simulink model "LW_ctrl_241029_1"  (R2024b)
settings: Solver=ode4  StartTime=0.0  StopTime=inf  FixedStep=0.005  RelTol=1e-3  EnableMultiTasking=on
StartFcn:
  | %timestart = cputime;
StopFcn:
  | %dt = cputime - timestart
undefined symbols (not defined in the file or in its folder): AttCtrl_cycle, ControlMode, DEG2RAD, Earth, FlightMode, LW_ACRO_P_MAX, LW_ACRO_R_MAX, LW_ACRO_Y_MAX, LW_AERO_C0, LW_AERO_C1, LW_AERO_Y0, LW_ANGLE, LW_DMZ0, LW_DMZ_MIN, LW_LAT_CIRCLE, LW_MAN_PITCH_MAX, LW_MAN_ROLL_MAX, LW_MASS, LW_OB_CIRCLE_R, LW_OB_CIRCLE_V, LW_OB_CIRCLE_W, LW_OB_TYPE, LW_REX_YAW, LW_SERVOL_MAX, LW_SERVOR_MAX, LW_TEST_DTXY, LW_TEST_DTZ, LW_THR_HOVER, LW_WZ_MAX, LW_X_ACCEL_MAX, LW_X_ACCEL_MIN, LW_X_FF, LW_X_JERK_MAX, LW_X_P, LW_X_VEL_MAX, LW_Y_ACCEL_MAX, LW_Y_ACCEL_MIN, LW_Y_FF, LW_Y_JERK_MAX, LW_Y_P, LW_Y_VEL_MAX, LW_YAW_KAD, LW_YAW_KAP, LW_Z_ACCEL_LOW, LW_Z_ACCEL_UP, LW_Z_FF, LW_Z_JERK_MAX, LW_Z_P, LW_Z_VEL_MAX_UP, Map_xoffset, Map_yoffset, Map_zoffset, MAX_wdotx, MAX_wdoty, MAX_wdotz, Mixer_cycle, ModelParam_AccelMax, ModelParam_DelayAtt, ModelParam_DelayOmega, ModelParam_DelayPos ... (+59)
libraries: pixhawk_slib_uORB_RW x15, simulink x7, slpidlib x6, dspfdesign x6, dspstat3 x5, aerolibnav x4, pixhawk_slib_sensors_actuators x3, aerolibtransform2 x3, etargetslib x2, pixhawk_slib_rfly x1, aerolibatmos2 x1, slrealtimeiplib x1
(part 1 of 6)
Description:
  | 20241104
  | 1.加入PX4中weather vane方法，并可以与偏航导纳相互切换，用于对比实验。
  | 2.加入没有进入定点以及手动控制偏航时对偏航导纳期望进行重置。
  |   进行了实飞测试，结果正常。
  | 
  | 20241030
  | 1.增加偏航导纳控制，加入4个偏航导纳控制相关的可调参数，并进行仿真测试。
  |   将力矩扰动估计放到状态更新模块中。
  | 2.修改模型加入φ理论气动力矩。
  | 3.位置控制输出部分增加姿态角速率，并在角速率控制部分加入手动模式下位置控制角速率前馈。
  | 20240905
  | 1.舵面滤波，增加舵面高速时的权重
  | 20240831
  | 1.加入舵面参数辨识的代码，修改混控制部分输出。
  |   设置参数为不使用舵面，在进入平飞状态时给一个固定的舵面角度。
  | 2.增加更多的直线轨迹，目前包括3,6,10,12,13,14,15,16,17,18,20
  | 20240826
  | 1.加入状态重置处理，包括控制器中、扰动估计中、offboard中
  | 2.修改混控器权重系数，优化空速较小时舵面变化大的问题。
  |   加入分别计算舵面和旋翼的代码。
  | 3.在6C和Pixhawk4中进行了实时性测试，250Hz都能实时运行；400Hz6C可以。
  | 
  | 关闭遥控器失联的处理；
  | 关闭acro模式；
  | 加入前馈系数；
  | 内置传感器中加入tfsensor启动指令；--20221019
  | 
  | 修改姿态控制逻辑，姿态误差在body系下求取，得到期望角速度之后转到lifting wing frame。--20221022
settings Model: Creator=Mr Wang  LastModifiedBy=bhcxq
settings SolverCC: AlgebraicLoopSolver=TrustRegion  PositivePriorityOrder=on  AutoInsertRateTranBlk=on
settings DataIOCC: ReturnWorkspaceOutputs=off
settings OptimizationCC: DefaultParameterBehavior=Inlined  MemcpyThreshold=128  MaxStackSize=128  EfficientTunableParamExpr=on
settings DebuggingCC: MergeDetectMultiDrivingBlocksExec=none  MultiTaskCondExecSysMsg=none  ParameterTunabilityLossMsg=error  UnconnectedInputMsg=warning  UnconnectedOutputMsg=warning  UnconnectedLineMsg=warning  AssertControl=DisableAll  ArithmeticOperatorsInVariantConditions=warning
settings HardwareCC: ProdBitPerPointer=32  ProdBitPerSizeT=32  ProdBitPerPtrDiffT=32  ProdLargestAtomicInteger=Long  ProdLargestAtomicFloat=Double  ProdWordSize=32  ProdHWDeviceType=ARM Compatible->ARM Cortex
settings ModelReferenceCC: EnableRefExpFcnMdlSchedulingChecks=on
settings SFSimCC: SimUseLocalCustomCode=off  MATLABDynamicMemAlloc=off  CustomCodeUndefinedFunction=UseInterfaceOnly
settings RTWCC: Description=Embedded Coder  SystemTargetFile=ert.tlc  HardwareBoard=Pixhawk PX4  TLCOptions="-aInlineSetEventsForThisBaseRateFcn=TLC_FALSE -aSuppressMultiTaskScheduler=TLC_FALSE  -aRateBasedStepFcn=0"  TemplateMakefile=ert_default_tmf  GenerateReport=on  RTWUseLocalCustomCode=off  CustomSource=px4_simulink_app_params.c  Toolchain=Pixhawk Toolchain  IncludeHyperlinkInReport=on  LaunchReport=on  CodeExecutionProfiling=on  CodeProfilingInstrumentation=detailed  GenerateTraceInfo=on  GenerateTraceReport=on  GenerateTraceReportSl=on  GenerateTraceReportSf=on  GenerateTraceReportEml=on  GPUComputeCapability=3.5  DLArmComputeVersion=19.05
settings CodeAppCC: ForceParamTrailComments=on  IgnoreCustomStorageClasses=off  OperatorAnnotations=on  SimulinkDataObjDesc=on  SFDataObjDesc=on  MATLABFcnDesc=on  InsertBlockDesc=on  StateflowObjectComments=on  MATLABSourceComments=on
settings ERTTargetCC: MultiwordLength=2048  SupportContinuousTime=on  SupportVariableSizeSignals=on  ExtModeTransport=1  ExtModeMexFile=ext_serial_win32_comm  ExtModeMexArgs=1 3 115200 10  InlinedParameterPlacement=Hierarchical  ERTCustomFileTemplate=px4_codertarget_file_process.tlc  ConvertIfToSwitch=off  DynamicArrayContainerType=coder::array
settings ConfigComp: PSEnableModelRefIgnoreList=off  PSModelRefMinMaxVerif=CheckAndConstrain  PSAutoStubLUT=on

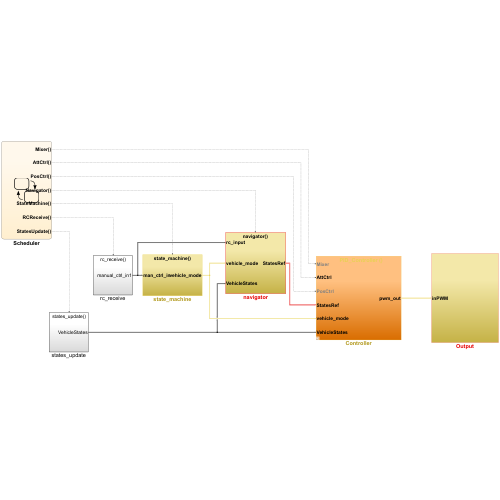
[thumbnail: Simulink's stored preview of the top-level diagram]
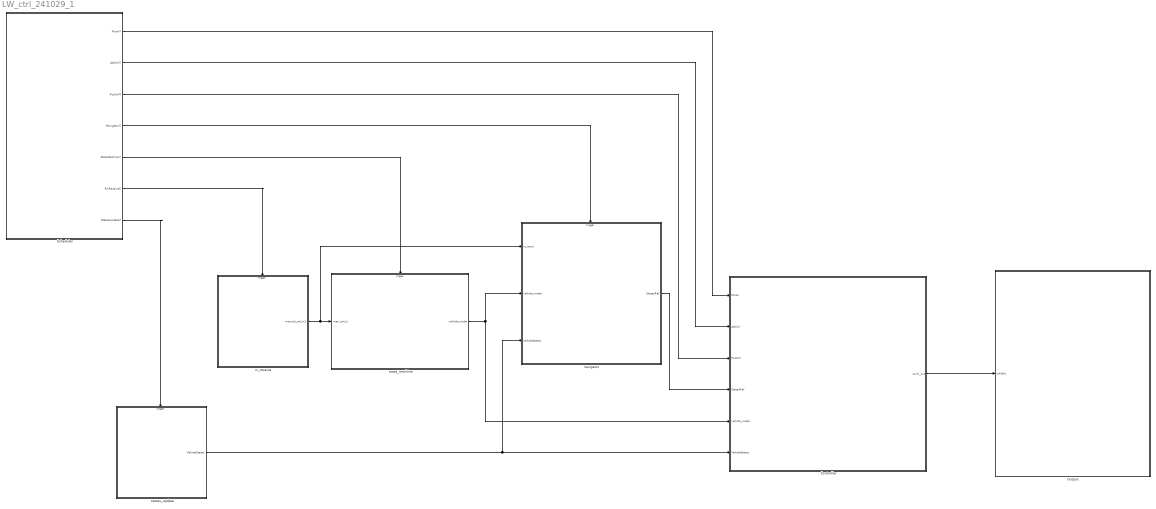
== system LW_ctrl_241029_1 ==
  Controller : Subsystem  Variant=on
  Output : Subsystem  Priority=8
  Scheduler : Stateflow chart  Priority=1  TreatAsAtomicUnit=on
  navigator : Subsystem  Priority=5
  rc_receive : Subsystem  Priority=3
  state_machine : Subsystem  Priority=4
  states_update : Subsystem  Priority=2
  wires:
  state_machine/1(vehicle_mode) -> Controller/5(vehicle_mode), navigator/2(vehicle_mode)
  rc_receive/1(manual_ctrl_in1) -> state_machine/1(man_ctrl_in), navigator/1(rc_input)
  states_update/1(VehicleStates) -> Controller/6(VehicleStates), navigator/3(VehicleStates)
  Scheduler/1(Mixer()) -> Controller/1(Mixer)
  Scheduler/2(AttCtrl()) -> Controller/2(AttCtrl)
  Scheduler/3(PosCtrl()) -> Controller/3(PosCtrl)
  Scheduler/7(StatesUpdate()) -> states_update/Trigger
  Scheduler/6(RCReceive()) -> rc_receive/Trigger
  Scheduler/5(StateMachine()) -> state_machine/Trigger
  Scheduler/4(Navigator()) -> navigator/Trigger
  navigator/1(StatesRef) -> Controller/4(StatesRef)
  Controller/1(pwm_out) -> Output/1(inPWM)

== system LW_ctrl_241029_1/Controller ==
  note: 1) Add Subsystem or Model blocks as valid variant choices.
      | 2) You cannot connect blocks at this level. At simulation, connectivity is automatically
      | determined, based on the active variant and port name matching.
  Mixer : Inport
  AttCtrl : Inport  Port=2
  PosCtrl : Inport  Port=3
  StatesRef : Inport  Port=4
  vehicle_mode : Inport  Port=5
  VehicleStates : Inport  Port=6
  PID_Controller : Subsystem  VariantControl=Controller_Switch <= 0.5
  pwm_out : Outport

== system LW_ctrl_241029_1/Output ==
  inPWM : Inport
  OutputSelect : Subsystem  Variant=on
  wires:
  inPWM/1 -> OutputSelect/1(inPWM)

== system LW_ctrl_241029_1/navigator ==
  rc_input : Inport
  vehicle_mode : Inport  Port=2
  VehicleStates : Inport  Port=3
  navigator : TriggerPort  TriggerType=function-call  VariantControl=Variant
  Bus Selector : BusSelector  OutputSignals=flight_mode
  StatesRefBus : BusCreator  Inputs=2
  Switch Case : SwitchCase  CaseConditions={FlightMode.PILOT, FlightMode.AUTO, FlightMode.OFFBOARD}  ShowDefaultCase=off
  Terminator : Terminator
  Terminator1 : Terminator
  logger : Subsystem  Variant=on
  navigator_manual : Subsystem  TreatAsAtomicUnit=on
  navigator_offboard : Subsystem  TreatAsAtomicUnit=on
  StatesRef : Outport  VectorParamsAs1DForOutWhenUnconnected=off
  tag scope: log_n_manual_ref=global, log_n_offboard_ref=global
  wires:
  Bus Selector/1 -> navigator_offboard/2(flight_mode), Switch Case/1  "<flight_mode>"
  Switch Case/1 -> navigator_manual/Action
  rc_input/1 -> navigator_offboard/3(RC_input), navigator_manual/1(rc_input)
  navigator_offboard/1(offboard_ref) -> [log_n_offboard_ref], StatesRefBus/2  "offboard"
  navigator_manual/1(manual_ref) -> [log_n_manual_ref], StatesRefBus/1  "manual"
  vehicle_mode/1 -> Bus Selector/1  "vehicle_mode"
  VehicleStates/1 -> navigator_offboard/1(VehicleStates)
  Switch Case/2 -> Terminator/1
  Switch Case/3 -> Terminator1/1
  StatesRefBus/1 -> StatesRef/1

== system LW_ctrl_241029_1/rc_receive ==
  rc_receive : TriggerPort  TriggerType=function-call  VariantControl=Variant
  manual_ctrl_in : Subsystem  Variant=on
  manual_ctrl_in1 : Outport
  wires:
  manual_ctrl_in/1(manual_ctrl_in) -> manual_ctrl_in1/1

== system LW_ctrl_241029_1/state_machine ==
  man_ctrl_in : Inport
  state_machine : TriggerPort  TriggerType=function-call  VariantControl=Variant
  Bus Creator : BusCreator  Inputs=3
  Bus Selector : BusSelector  OutputSignals=AU8,RC_Lost,AU5,AU7,AU6
  Bus Selector1 : BusSelector  OutputSignals=armed
  MATLAB Function3 : MATLAB Function  TreatAsAtomicUnit=on
  MATLAB Function4 : MATLAB Function  TreatAsAtomicUnit=on
  logger : Subsystem  Variant=on
  uORB Read Function-Call Trigger : pixhawk_slib_uORB_RW/uORB Read Function-Call Trigger  uORB_Topic_str='actuator_armed'  BusObjVar=Bus: actuator_armed_SL  uORB_Interval=4  AsyncOutput=off  Fcn_call_select=Generate Function Call Signal  TaskName='Task1'  Poll_timeout=-1  Ts=-1
      settings: SourceProductName=uORB Read / Write Blocks
  vehicle_mode : Outport  VectorParamsAs1DForOutWhenUnconnected=off
  tag scope: log_sm_vehicle_mode=global
  wires:
  man_ctrl_in/1 -> Bus Selector/1
  Bus Selector/3 -> MATLAB Function4/1(ch5)  "<AU5>"
  Bus Selector/2 -> MATLAB Function4/4(RC_Lost)  "<RC_Lost>"
  MATLAB Function4/2(flight_mode) -> Bus Creator/1
  Bus Selector/4 -> MATLAB Function4/2(ch7)  "<AU7>"
  Bus Selector/5 -> MATLAB Function3/1(ch6)  "<AU6>"
  Bus Creator/1 -> [log_sm_vehicle_mode], vehicle_mode/1
  MATLAB Function3/1(arm) -> Bus Creator/3  "arm"
  Bus Selector/1 -> MATLAB Function4/3(ch8)  "<AU8>"
  MATLAB Function4/1(ctrl_mode) -> Bus Creator/2  "ctrl_mode"
  uORB Read Function-Call Trigger/1 -> Bus Selector1/1
  Bus Selector1/1 -> MATLAB Function3/2(armed), MATLAB Function4/5(armed)  "<armed>"

== system LW_ctrl_241029_1/states_update ==
  states_update : TriggerPort  TriggerType=function-call  VariantControl=Variant
  Bus Creator : BusCreator  Inputs=8
  vehicle_local_position : Subsystem  Variant=on
  VehicleStates : Outport
  wires:
  vehicle_local_position/3(vehicle_attitude) -> Bus Creator/3  "vehicle_attitude"
  vehicle_local_position/2(airspeed) -> Bus Creator/2  "airspeed"
  vehicle_local_position/1(vehicle_local_position) -> Bus Creator/1  "vehicle_local_position"
  Bus Creator/1 -> VehicleStates/1
  vehicle_local_position/4(vehicle_global_position) -> Bus Creator/4  "vehicle_global_position"
  vehicle_local_position/5(battery_status) -> Bus Creator/5  "battery_status"
  vehicle_local_position/6(T_limit) -> Bus Creator/6  "T_limit"
  vehicle_local_position/7(sensor_imu) -> Bus Creator/7  "sensor_imu"
  vehicle_local_position/8(states_flag) -> Bus Creator/8  "states_flag"

== system LW_ctrl_241029_1/Controller/PID_Controller ==
  StatesRef : Inport
  vehicle_mode : Inport  Port=2
  VehicleStates : Inport  Port=3
  AttCtrl : TriggerPort  TriggerType=function-call  VariantControl=Variant
  PID_Controller : Subsystem  VariantControl=Controller_Switch <= 1.5 && Controller_Switch >= 0.5
  pwm_out : Outport
  wires:
  StatesRef/1 -> PID_Controller/1(StatesRef)
  PID_Controller/1(pwm_out) -> pwm_out/1
  vehicle_mode/1 -> PID_Controller/2(vehicle_mode)
  VehicleStates/1 -> PID_Controller/3(VehicleStates)

== system LW_ctrl_241029_1/Output/OutputSelect ==
  note: 1) Add Subsystem or Model blocks as valid variant choices.
      | 2) You cannot connect blocks at this level. At simulation, connectivity is automatically
      | determined, based on the active variant and port name matching.
  inPWM : Inport
  FLY : Subsystem  VariantControl=VSS_PROCEDURE_FLY
  HIL : Subsystem  VariantControl=VSS_PROCEDURE_HIL
  Sim : Subsystem  TreatAsAtomicUnit=on  VariantControl=VSS_PROCEDURE_SIM

== system LW_ctrl_241029_1/navigator/logger ==
  HIL&FLY : Subsystem  VariantControl=VSS_PROCEDURE_HIL_FLY
  Sim : Subsystem  VariantControl=VSS_PROCEDURE_SIM

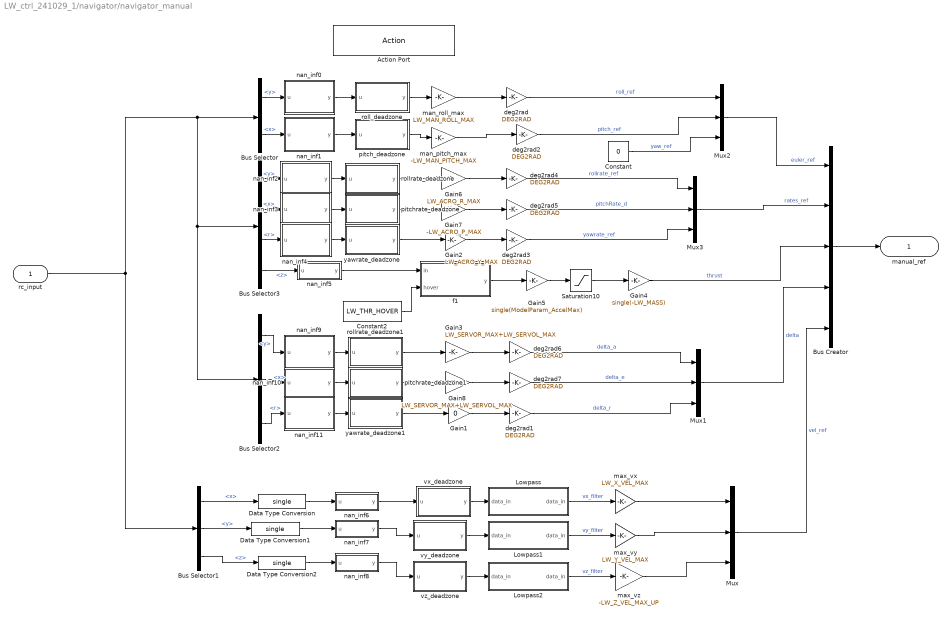
== system LW_ctrl_241029_1/navigator/navigator_manual ==
  rc_input : Inport
  Action Port : ActionPort  ActionPortLabel=case [ PILOT ]:
  Bus Creator : BusCreator  Inputs=5
  Bus Selector : BusSelector  OutputSignals=y,x
  Bus Selector1 : BusSelector  OutputSignals=x,y,z
  Bus Selector2 : BusSelector  OutputSignals=y,x,r
  Bus Selector3 : BusSelector  OutputSignals=y,x,r,z
  Constant : Constant  Value=0  OutDataTypeStr=single
  Constant2 : Constant  Value=LW_THR_HOVER
  Data Type Conversion : DataTypeConversion  OutDataTypeStr=single  SaturateOnIntegerOverflow=off  RndMeth=Floor
  Data Type Conversion1 : DataTypeConversion  OutDataTypeStr=single  SaturateOnIntegerOverflow=off  RndMeth=Floor
  Data Type Conversion2 : DataTypeConversion  OutDataTypeStr=single  SaturateOnIntegerOverflow=off  RndMeth=Floor
  Gain1 : Gain  Gain=0
  Gain2 : Gain  Gain=LW_ACRO_Y_MAX
  Gain3 : Gain  Gain=LW_SERVOR_MAX+LW_SERVOL_MAX  OutDataTypeStr=Inherit: Inherit via back propagation
  Gain4 : Gain  Gain=single(-LW_MASS)
  Gain5 : Gain  Gain=single(ModelParam_AccelMax)
  Gain6 : Gain  Gain=LW_ACRO_R_MAX  OutDataTypeStr=Inherit: Inherit via back propagation
  Gain7 : Gain  Gain=-LW_ACRO_P_MAX  OutDataTypeStr=Inherit: Inherit via back propagation
  Gain8 : Gain  Gain=LW_SERVOR_MAX+LW_SERVOL_MAX  OutDataTypeStr=Inherit: Inherit via back propagation
  Lowpass : MATLAB Function  TreatAsAtomicUnit=on
  Lowpass1 : MATLAB Function  TreatAsAtomicUnit=on
  Lowpass2 : MATLAB Function  TreatAsAtomicUnit=on
  Mux{,1..3} (4 alike) : Mux  Inputs=3
  Saturation10 : Saturate  UpperLimit=single(5+ModelParam_envGravityAcc)  LowerLimit=0
  deg2rad{,1..7} (8 alike) : Gain  Gain=DEG2RAD
  f1 : MATLAB Function  TreatAsAtomicUnit=on
  man_pitch_max : Gain  Gain=-LW_MAN_PITCH_MAX  OutDataTypeStr=Inherit: Inherit via back propagation
  man_roll_max : Gain  Gain=LW_MAN_ROLL_MAX  OutDataTypeStr=Inherit: Inherit via back propagation
  max_vx : Gain  Gain=LW_X_VEL_MAX  OutDataTypeStr=Inherit: Inherit via back propagation
  max_vy : Gain  Gain=LW_Y_VEL_MAX  OutDataTypeStr=Inherit: Inherit via back propagation
  max_vz : Gain  Gain=-LW_Z_VEL_MAX_UP  OutDataTypeStr=Inherit: Inherit via back propagation
  nan_inf0 : MATLAB Function  TreatAsAtomicUnit=on
  nan_inf1 : MATLAB Function  TreatAsAtomicUnit=on
  nan_inf10 : MATLAB Function  TreatAsAtomicUnit=on
  nan_inf11 : MATLAB Function  TreatAsAtomicUnit=on
  nan_inf2 : MATLAB Function  TreatAsAtomicUnit=on
  nan_inf3 : MATLAB Function  TreatAsAtomicUnit=on
  nan_inf4 : MATLAB Function  TreatAsAtomicUnit=on
  nan_inf5 : MATLAB Function  TreatAsAtomicUnit=on
  nan_inf6 : MATLAB Function  TreatAsAtomicUnit=on
  nan_inf7 : MATLAB Function  TreatAsAtomicUnit=on
  nan_inf8 : MATLAB Function  TreatAsAtomicUnit=on
  nan_inf9 : MATLAB Function  TreatAsAtomicUnit=on
  pitch_deadzone : MATLAB Function  TreatAsAtomicUnit=on
  pitchrate_deadzone : MATLAB Function  TreatAsAtomicUnit=on
  pitchrate_deadzone1 : MATLAB Function  TreatAsAtomicUnit=on
  roll_deadzone : MATLAB Function  TreatAsAtomicUnit=on
  rollrate_deadzone : MATLAB Function  TreatAsAtomicUnit=on
  rollrate_deadzone1 : MATLAB Function  TreatAsAtomicUnit=on
  vx_deadzone : MATLAB Function  TreatAsAtomicUnit=on
  vy_deadzone : MATLAB Function  TreatAsAtomicUnit=on
  vz_deadzone : MATLAB Function  TreatAsAtomicUnit=on
  yawrate_deadzone : MATLAB Function  TreatAsAtomicUnit=on
  yawrate_deadzone1 : MATLAB Function  TreatAsAtomicUnit=on
  manual_ref : Outport
  wires:
  Gain4/1 -> Bus Creator/3  "thrust"
  man_roll_max/1 -> deg2rad/1
  Gain2/1 -> deg2rad3/1
  man_pitch_max/1 -> deg2rad2/1
  Bus Creator/1 -> manual_ref/1
  Bus Selector3/3 -> nan_inf4/1(u)  "<r>"
  deg2rad/1 -> Mux2/1  "roll_ref"
  Bus Selector3/4 -> nan_inf5/1(u)  "<z>"
  deg2rad2/1 -> Mux2/2  "pitch_ref"
  Bus Selector/2 -> nan_inf1/1(u)  "<x>"
  Bus Selector/1 -> nan_inf0/1(u)  "<y>"
  deg2rad3/1 -> Mux3/3  "yawrate_ref"
  Bus Selector1/3 -> Data Type Conversion2/1  "<z>"
  Data Type Conversion/1 -> nan_inf6/1(u)
  Data Type Conversion2/1 -> nan_inf8/1(u)
  Bus Selector1/2 -> Data Type Conversion1/1  "<y>"
  Data Type Conversion1/1 -> nan_inf7/1(u)
  Bus Selector1/1 -> Data Type Conversion/1  "<x>"
  max_vz/1 -> Mux/3
  max_vx/1 -> Mux/1
  max_vy/1 -> Mux/2
  Mux/1 -> Bus Creator/5  "vel_ref"
  Constant/1 -> Mux2/3  "yaw_ref"
  Mux2/1 -> Bus Creator/1  "euler_ref"
  deg2rad4/1 -> Mux3/1  "rollrate_ref"
  Gain6/1 -> deg2rad4/1
  Bus Selector3/1 -> nan_inf2/1(u)  "<y>"
  deg2rad5/1 -> Mux3/2  "pitchRate_d"
  Gain7/1 -> deg2rad5/1
  Bus Selector3/2 -> nan_inf3/1(u)  "<x>"
  Mux3/1 -> Bus Creator/2  "rates_ref"
  nan_inf5/1(y) -> f1/1(in)
  Gain5/1 -> Saturation10/1
  Saturation10/1 -> Gain4/1
  roll_deadzone/1(y) -> man_roll_max/1
  pitch_deadzone/1(y) -> man_pitch_max/1
  rollrate_deadzone/1(y) -> Gain6/1
  pitchrate_deadzone/1(y) -> Gain7/1
  yawrate_deadzone/1(y) -> Gain2/1
  vx_deadzone/1(y) -> Lowpass/1("data_in ")
  vy_deadzone/1(y) -> Lowpass1/1("data_in ")
  vz_deadzone/1(y) -> Lowpass2/1("data_in ")
  nan_inf0/1(y) -> roll_deadzone/1(u)
  nan_inf1/1(y) -> pitch_deadzone/1(u)
  nan_inf2/1(y) -> rollrate_deadzone/1(u)
  nan_inf3/1(y) -> pitchrate_deadzone/1(u)
  nan_inf4/1(y) -> yawrate_deadzone/1(u)
  nan_inf6/1(y) -> vx_deadzone/1(u)
  nan_inf7/1(y) -> vy_deadzone/1(u)
  nan_inf8/1(y) -> vz_deadzone/1(u)
  f1/1(y) -> Gain5/1
  Constant2/1 -> f1/2(hover)
  nan_inf11/1(y) -> yawrate_deadzone1/1(u)
  nan_inf10/1(y) -> pitchrate_deadzone1/1(u)
  nan_inf9/1(y) -> rollrate_deadzone1/1(u)
  yawrate_deadzone1/1(y) -> Gain1/1
  pitchrate_deadzone1/1(y) -> Gain8/1
  rollrate_deadzone1/1(y) -> Gain3/1
  Mux1/1 -> Bus Creator/4  "delta"
  Bus Selector2/2 -> nan_inf10/1(u)  "<x>"
  Gain8/1 -> deg2rad7/1
  deg2rad7/1 -> Mux1/2  "delta_e"
  Bus Selector2/1 -> nan_inf9/1(u)  "<y>"
  Gain3/1 -> deg2rad6/1
  deg2rad6/1 -> Mux1/1  "delta_a"
  deg2rad1/1 -> Mux1/3  "delta_r"
  Bus Selector2/3 -> nan_inf11/1(u)  "<r>"
  Gain1/1 -> deg2rad1/1
  rc_input/1 -> Bus Selector1/1, Bus Selector2/1, Bus Selector3/1, Bus Selector/1
  Lowpass/1(data_in) -> max_vx/1  "vx_filter"
  Lowpass1/1(data_in) -> max_vy/1  "vy_filter"
  Lowpass2/1(data_in) -> max_vz/1  "vz_filter"

== system LW_ctrl_241029_1/navigator/navigator_offboard ==
  VehicleStates : Inport
  flight_mode : Inport  Port=2
  RC_input : Inport  Port=3
  Bus Selector1 : BusSelector  OutputSignals=AU8
  Bus Selector2 : BusSelector  OutputSignals=vehicle_local_position.timestamp,vehicle_local_position.vehicle_local_pos,vehicle_local_position.vehicle_local_vel,vehicle_attitude.quat,airspeed.v_wind
  Data Type Conversion : DataTypeConversion  OutDataTypeStr=single  SaturateOnIntegerOverflow=off  RndMeth=Floor
  Gain : Gain  Gain=1.0e-6
  task select : Subsystem
  offboard_ref : Outport  OutDataTypeStr=Bus: offboard_bus
  wires:
  Bus Selector2/2 -> task select/3(pos)  "<vehicle_local_pos>"
  Bus Selector2/3 -> task select/4(vel)  "<vehicle_local_vel>"
  Bus Selector2/4 -> task select/5(q)  "<quat>"
  Data Type Conversion/1 -> task select/1(timestamp)
  VehicleStates/1 -> Bus Selector2/1
  flight_mode/1 -> task select/2(flight_mode)
  Gain/1 -> Data Type Conversion/1
  Bus Selector2/5 -> task select/7(v_wind)  "<v_wind>"
  Bus Selector2/1 -> Gain/1  "<timestamp>"
  RC_input/1 -> Bus Selector1/1
  Bus Selector1/1 -> task select/6(CH8)  "<AU8>"
  task select/1(offboard_ref) -> offboard_ref/1

== system LW_ctrl_241029_1/rc_receive/manual_ctrl_in ==
  HIL&FLY V1.13.3 : Subsystem  VariantControl=VSS_PROCEDURE_HIL_FLY_V1_13
  Sim : Subsystem  VariantControl=VSS_PROCEDURE_SIM
  manual_ctrl_in : Outport  VectorParamsAs1DForOutWhenUnconnected=off

== system LW_ctrl_241029_1/state_machine/logger ==
  HIL&FLY : Subsystem  VariantControl=VSS_PROCEDURE_HIL_FLY
  Sim : Subsystem  VariantControl=VSS_PROCEDURE_SIM

== system LW_ctrl_241029_1/states_update/vehicle_local_position ==
  HIL&FLY V1.13.3 : Subsystem  VariantControl=VSS_PROCEDURE_HIL_FLY_V1_13
  Sim : Subsystem  VariantControl=VSS_PROCEDURE_SIM
  vehicle_local_position : Outport  VectorParamsAs1DForOutWhenUnconnected=off
  airspeed : Outport  Port=2  VectorParamsAs1DForOutWhenUnconnected=off
  vehicle_attitude : Outport  Port=3  VectorParamsAs1DForOutWhenUnconnected=off
  vehicle_global_position : Outport  Port=4  OutDataTypeStr=Bus: vehicle_global_position_bus  VectorParamsAs1DForOutWhenUnconnected=off
  battery_status : Outport  Port=5  OutDataTypeStr=Bus: battery_status_bus  VectorParamsAs1DForOutWhenUnconnected=off
  T_limit : Outport  Port=6  VectorParamsAs1DForOutWhenUnconnected=off
  sensor_imu : Outport  Port=7  VectorParamsAs1DForOutWhenUnconnected=off
  states_flag : Outport  Port=8  VectorParamsAs1DForOutWhenUnconnected=off

== system LW_ctrl_241029_1/Controller/PID_Controller/PID_Controller ==
  StatesRef : Inport
  vehicle_mode : Inport  Port=2
  VehicleStates : Inport  Port=3
  Bus Creator : BusCreator  Inputs=2
  Bus Selector : BusSelector  OutputSignals=arm
  Compare To Constant : simulink/Logic and Bit Operations/Compare To Constant  relop===  const=ControlMode.ARM  OutDataTypeStr=boolean
  Constant1 : Constant  Value=single([ones(4,1)*900;ones(4,1)*1500])
  Constant2 : Constant  Value=single([ones(4,1)*1500])
  Mux1 : Mux  Inputs=2
  Saturation : Saturate  UpperLimit=[2000 2000 2000 2000 2000 2000 2000 2000]  LowerLimit=[1000 1000 1000 1000 1000 1000 0 1000]
  Switch : Switch  Criteria=u2 ~= 0  SaturateOnIntegerOverflow=off  InputSameDT=off
  altitude control : Subsystem
  local_pos_ref_selector : Subsystem
      settings: PortSchema="{\"entries\":[{\"content\":{\"sides\":[{\"content\":{\"connectorIds\":[\"In1\",\"In2\"]},\"type\":\"ConnectorPlacement.EquallySpacedRectSide\",\"uuid\":\"af9e33bb-35de-42c3-af2d-f6d503a747ed\"},{\"content\":{\"connectorIds\":[\"Out1\"],\"side\":\"RIGHT\"},\"type\":\"ConnectorPlacement.EquallySpacedRectSide\",\"uuid\":\"523d2ad7-493f-4e71-872f-c007353d3e53\"},{\"content\":{\"connectorIds\":[\"In3\"],\"side\":\"TOP\"},\"type\":\"ConnectorPlacement.EquallySpacedRectSide\",\"uuid\":\"8a55ba44-5970-453a-95a4-1a368c892611\"},{\"content\":{\"connectorIds\":[],\"side\":\"BOTTOM\"},\"type\":\"ConnectorPlacement.EquallySpacedRectSide\",\"uuid\":\"56716612-c0a6-4d29-908f-4ac693186525\"}]},\"type\":\"ConnectorPlacement.EquallySpacedConnector\",\"uuid\":\"ec9a3631-cdf0-459e-8e4d-c728b4850c15\"}],\"packageUris\":[\"http://schema.mathworks.com/mf0/Connector/R2020b\"],\"version\":\"1.0\"}"
  nan_inf_mode : MATLAB Function  TreatAsAtomicUnit=on
  postion control : Subsystem
  select parameter : Subsystem
  toPWM : Subsystem
  pwm_out : Outport
  wires:
  Bus Creator/1 -> pwm_out/1
  select parameter/1(theta) -> postion control/4(theta)
  select parameter/2(phi) -> postion control/3(phi)
  select parameter/3(wx) -> altitude control/1(p)
  select parameter/4(wy) -> altitude control/2(q)
  postion control/1(attitude_d) -> altitude control/3(attitude_d)
  select parameter/5(wz) -> altitude control/4(r)
  postion control/2(f_d) -> altitude control/5(f_d)
  select parameter/7(quat) -> altitude control/6(quat)
  local_pos_ref_selector/1(local_pos_ref) -> postion control/2(local_pos_ref)
  select parameter/6(psi) -> postion control/5(psi)
  StatesRef/1 -> local_pos_ref_selector/1(StatesRef)
  vehicle_mode/1 -> local_pos_ref_selector/2(vehicle_mode), postion control/6(Vehiclemode), Bus Selector/1, altitude control/7(vehicle_mode)
  VehicleStates/1 -> postion control/1(VehicleStates), local_pos_ref_selector/3(VehicleStates), select parameter/1(VehicleStates), toPWM/2(voltage)
  Saturation/1 -> Bus Creator/2  "pwm"
  Switch/1 -> Saturation/1
  Compare To Constant/1 -> Switch/2
  altitude control/1(T) -> toPWM/1(T)
  Mux1/1 -> Switch/1
  Constant1/1 -> Switch/3
  nan_inf_mode/1(y) -> Bus Creator/1, Compare To Constant/1  "arm"
  Bus Selector/1 -> nan_inf_mode/1(u)  "<arm>"
  Constant2/1 -> Mux1/2
  toPWM/1(pwm) -> Mux1/1

== system LW_ctrl_241029_1/Output/OutputSelect/FLY ==
  inPWM : Inport
  Bus Selector : BusSelector  OutputSignals=arm,pwm
  Compare To Constant : simulink/Logic and Bit Operations/Compare To Constant  relop===  const=ControlMode.ARM  OutDataTypeStr=boolean
  Data Type Conversion2 : DataTypeConversion  OutDataTypeStr=uint16  SaturateOnIntegerOverflow=off  RndMeth=Floor
  Demux : Demux  Outputs=6
  PWM_output : pixhawk_slib_sensors_actuators/PWM_output  Description=|  pub_outputs=on  pwm_rate=400Hz  show_pwm1=on  show_pwm5=on  show_pwm2=on  show_pwm6=on  show_pwm3=on  show_pwm7=off  show_pwm4=on  show_pwm8=off
      | This block allows the user to send the appropriate PWM signals out to the PX4 outputs.  
      | These are usually connected to the ESCs which control the motor speeds. 
      | In order for the flight control to arm (enable) the output from the software side, the ARM Output input must be held high (boolean TRUE).  
      | Only then will the PWM values be sent out the PX4 hardware ports.  
      | This is usually a function of the RC Tx in combination with other flight modes programmed in the Simulink model by the user.  
      | The block has 8 available ports (data type uint16) which can be selectively chosen.  
      | These correspond to the 8 PWM output ports on the px4fmu hardware.
      settings: SourceProductName=Sensors and Actuators
  Selector1 : Selector  InputPortWidth=8  IndexOptions=Index vector (dialog)  Indices=[1:6]  OutputSizes=1
  wires:
  Compare To Constant/1 -> PWM_output/1
  Selector1/1 -> Data Type Conversion2/1
  Demux/1 -> PWM_output/2
  Demux/3 -> PWM_output/4
  inPWM/1 -> Bus Selector/1
  Bus Selector/1 -> Compare To Constant/1  "<arm>"
  Bus Selector/2 -> Selector1/1  "<pwm>"
  Demux/5 -> PWM_output/6  "er"
  Demux/6 -> PWM_output/7  "el"
  Data Type Conversion2/1 -> Demux/1
  Demux/2 -> PWM_output/3
  Demux/4 -> PWM_output/5

== system LW_ctrl_241029_1/Output/OutputSelect/HIL ==
  note: 16维输出
  inPWM : Inport
  Bus Selector : BusSelector  OutputSignals=pwm
  Constant : Constant  Value=zeros(1,8)
  Data Type Conversion : DataTypeConversion  OutDataTypeStr=single  SaturateOnIntegerOverflow=off  RndMeth=Floor
  Data Type Conversion2 : DataTypeConversion  OutDataTypeStr=single  SaturateOnIntegerOverflow=off  RndMeth=Floor
  HIL16CtrlsPWM : pixhawk_slib_rfly/HIL16CtrlsPWM  isAutoArm=off  isAutoBlock=on  isAutoLoiter=off  SamTime=-1
      settings: SourceProductName=RflySim APIs
  MATLAB Function : MATLAB Function  TreatAsAtomicUnit=on
  MATLAB Function1 : MATLAB Function  TreatAsAtomicUnit=on
  MATLAB Function2 : MATLAB Function  TreatAsAtomicUnit=on
  Mux : Mux  Inputs=2
  Terminator : Terminator
  input_rc : pixhawk_slib_sensors_actuators/input_rc  Description=|  sampletime=-1  channel1=off  channel2=off  channel3=off  channel4=off  channel5=on  channel6=off  channel7=off  channel8=off  channel9=off  channel10=off  channel11=off  channel12=off  channel13=off  channel14=off  channel15=off  channel16=off  channel17=off  channel18=off  ch_count=off  rssi=off  rc_failsafe=off  rc_lost=off  rc_inputsource=off
      | RC Input Block
      | 
      | This block provides user input control to the model.
      | It uses the input_rc uORB topic.
      | 
      | The user has the ability to choose which channels are available as outputs from this block and also some optional outputs. These include 
      | Channels 1 through 18
      | double data type indicating the PWM value from the controller 
      | measured pulse widths for each of the supported channels 
      | Channel Count 
      | uint32 data type of the number of channels which are detector by the PX4 
      | RC Failsafe 
      | boolean data types indicating that the RC Tx is sending the FailSafe signal (if equipped and properly setup) 
      | explicit failsafe flag: true on TX failure or TX out of range , false otherwise. 
      | Only the true state is reliable, as there are some (PPM) receivers on the market going into failsafe without telling us explicitly. 
      | RC Input Source 
      | Enumeration data type indicating which source the RC input is from. 
      | Valid values are found in the ENUM file: RC_INPUT_SOURCE_ENUM.m 
      |           Enumeration members for class 'RC_INPUT_SOURCE_ENUM':
      |           RCINPUT_SOURCE_UNKNOWN         (0)
      |           RCINPUT_SOURCE_PX4FMU_PPM      (1)
      |           RCINPUT_SOURCE_PX4IO_PPM       (2)
      |           RCINPUT_SOURCE_PX4IO_SPEKTRUM  (3)
      |           RCINPUT_SOURCE_PX4IO_SBUS      (4)
      |           RCINPUT_SOURCE_PX4IO_ST24      (5)
      |           RCINPUT_SOURCE_MAVLINK         (6)
      |           RCINPUT_SOURCE_QURT            (7)
      |           RCINPUT_SOURCE_PX4FMU_SPEKTRUM (8)
      |           RCINPUT_SOURCE_PX4FMU_SBUS     (9)
      |           RCINPUT_SOURCE_PX4FMU_ST24     (10)
      |           RCINPUT_SOURCE_PX4FMU_SUMD     (11)
      |           RCINPUT_SOURCE_PX4FMU_DSM      (12)
      |           RCINPUT_SOURCE_PX4IO_SUMD      (13)
      | 
      | RSSI - Receive signal strength index 
      | receive signal strength indicator (RSSI): < 0: Undefined, 0: no signal, 255: full reception 
      | RC Lost Connection 
      | boolean data type indicating RC receiver connection status 
      | True, if no frame has arrived in the expected time, false otherwise. 
      | True usally means that the receiver has been disconnected, but can also indicate a radio link loss on "stupid" systems. 
      | Will remain false, if a RX with failsafe option continues to transmit frames after a link loss. 
      |   
      | Sample Model: px4demo_input_rc.slx
      settings: SourceProductName=Sensors and Actuators
  uORB Write Advanced : pixhawk_slib_uORB_RW/uORB Write Advanced  Commented=on  Ts=0  uORB_AdvtQueue=on  uORB_FieldEnabledArr="0  0  0  1  0  0  0  0  0  0  0"  uORB_Topic_str=0  uORB_Struct_DT="[1  1  1  1  1]"  BlockInputCount=5  uORB_StructParams="[\"voltage_v\",\"voltage_filtered_v\",\"current_a\",\"current_filtered_a\",\"remaining\"]"  uORB_PortSizes="[1  1  1  1]"  MsgSizeOf=0  MW_update=true
      settings: SourceProductName=uORB Read / Write Blocks
  wires:
  inPWM/1 -> Bus Selector/1
  Data Type Conversion2/1 -> Mux/1
  Constant/1 -> Data Type Conversion/1
  Data Type Conversion/1 -> Mux/2
  input_rc/1 -> MATLAB Function/1(u)
  MATLAB Function/1(y) -> HIL16CtrlsPWM/1
  Mux/1 -> HIL16CtrlsPWM/2, uORB Write Advanced/1
  MATLAB Function1/1(y) -> Data Type Conversion2/1
  MATLAB Function2/1(out) -> Terminator/1
  Bus Selector/1 -> MATLAB Function1/1(u)  "<pwm>"

== system LW_ctrl_241029_1/Output/OutputSelect/Sim ==
  inPWM : Inport
  Bus Selector : BusSelector  OutputSignals=pwm,arm
  Compare To Constant : simulink/Logic and Bit Operations/Compare To Constant  relop===  const=ControlMode.ARM  OutDataTypeStr=boolean
  Compare To Constant1 : simulink/Logic and Bit Operations/Compare To Constant  relop=>=  const=0.2  OutDataTypeStr=boolean
  Constant1 : Constant  Value=single([ones(4,1)*1000;ones(4,1)*1500])
  DISARM : Constant  Value=ControlMode.DISARM
  Data Type Conversion : DataTypeConversion  OutDataTypeStr=double  SaturateOnIntegerOverflow=off  RndMeth=Floor
  Digital Clock : DigitalClock  SampleTime=0.001
  Lifting Body Airframe : Subsystem  InitFcn=|
      | ModelParam_servoT = 0.02; %1/(Ts+1)
      | ModelParam_servoCr = pi/2; %(-1,1)->(-pi/2,pi/2) 
      | ModelParam_LBCY = 0.0; %
      | ModelParam_LBCn = 0; %偏航力矩系数
      | ModelParam_LBCn_d = 0; %偏航舵操纵导数
      | ModelInit_servoRads = 0; %Init servo angle(rad)
  Switch : Switch  Criteria=u2 ~= 0  SaturateOnIntegerOverflow=off  InputSameDT=off
  Switch1 : Switch  Criteria=u2 > Threshold  SaturateOnIntegerOverflow=off  InputSameDT=off
  nan_inf : MATLAB Function  TreatAsAtomicUnit=on
  wires:
  inPWM/1 -> Bus Selector/1
  Data Type Conversion/1 -> Lifting Body Airframe/1(inPWM)
  nan_inf/1(y) -> Data Type Conversion/1
  Bus Selector/1 -> Switch/1  "<pwm>"
  Compare To Constant1/1 -> Switch1/2
  Digital Clock/1 -> Compare To Constant1/1
  DISARM/1 -> Switch1/3
  Bus Selector/2 -> Switch1/1  "<arm>"
  Compare To Constant/1 -> Switch/2
  Constant1/1 -> Switch/3
  Switch1/1 -> Compare To Constant/1  "arm"
  Switch/1 -> nan_inf/1(u)

== system LW_ctrl_241029_1/navigator/logger/HIL&FLY ==
  Data Type Conversion : DataTypeConversion  Priority=10  OutDataTypeStr=double  SaturateOnIntegerOverflow=off  RndMeth=Floor
  Data Type Conversion1 : DataTypeConversion  Priority=10  OutDataTypeStr=single  SaturateOnIntegerOverflow=off  RndMeth=Floor
  Data Type Conversion2 : DataTypeConversion  Priority=10  Commented=on  OutDataTypeStr=single  SaturateOnIntegerOverflow=off  RndMeth=Floor
  Data Type Conversion3 : DataTypeConversion  Priority=10  OutDataTypeStr=single  SaturateOnIntegerOverflow=off  RndMeth=Floor
  Data Type Conversion4 : DataTypeConversion  Priority=10  Commented=on  OutDataTypeStr=single  SaturateOnIntegerOverflow=off  RndMeth=Floor
  Data Type Conversion5 : DataTypeConversion  Priority=10  OutDataTypeStr=single  SaturateOnIntegerOverflow=off  RndMeth=Floor
  Demux : Demux  Outputs=[22,1]
  Mux : Mux  Inputs=2
  get_delta_t : Subsystem
  hrt_timestamp : MATLAB Function  TreatAsAtomicUnit=on
  log_n_missionInfo : From  Commented=on  GotoTag=log_n_missionInfo  TagVisibility=global
  log_n_non_manual_ref : From  Commented=on  GotoTag=log_n_non_manual_ref  TagVisibility=global
  uORB Write Advanced : pixhawk_slib_uORB_RW/uORB Write Advanced  Ts=0  uORB_AdvtQueue=on  uORB_FieldEnabledArr="0  0  0  1  0  0  0  0  0  0  0"  uORB_Topic_str=0  uORB_Struct_DT="[1  1  1  1  1]"  BlockInputCount=5  uORB_StructParams="[\"voltage_v\",\"voltage_filtered_v\",\"current_a\",\"current_filtered_a\",\"remaining\"]"  uORB_PortSizes="[1  1  1  1]"  MsgSizeOf=0  MW_update=true
      settings: SourceProductName=uORB Read / Write Blocks
  wires:
  hrt_timestamp/1(ts) -> Data Type Conversion/1
  Data Type Conversion/1 -> uORB Write Advanced/1, get_delta_t/1(timestamp)
  get_delta_t/1(delta_t) -> uORB Write Advanced/2
  [log_n_manual_ref] -> Data Type Conversion1/1
  log_n_non_manual_ref/1 -> Data Type Conversion2/1  "auto_ref"
  Data Type Conversion1/1 -> uORB Write Advanced/3
  log_n_missionInfo/1 -> Data Type Conversion4/1
  Data Type Conversion5/1 -> Mux/2
  Demux/1 -> Data Type Conversion3/1
  [log_n_offboard_ref] -> Demux/1  "offboard_ref"
  Demux/2 -> Data Type Conversion5/1
  Mux/1 -> uORB Write Advanced/4
  Data Type Conversion3/1 -> Mux/1

== system LW_ctrl_241029_1/navigator/logger/Sim ==
  Bus Creator : BusCreator  Inputs=2
  Bus Creator1 : BusCreator  Inputs=5
  Bus Creator2 : BusCreator  Inputs=10
  Bus Selector : BusSelector  OutputSignals=euler_ref,rates_ref,thrust,vel_ref,delta
  Bus Selector1 : BusSelector  OutputSignals=pos,vel,acc,q,f_d,alpha,beta,rates,dotrates,OB_TASK
  Data Type Conversion : DataTypeConversion  OutDataTypeStr=double  SaturateOnIntegerOverflow=off  RndMeth=Floor
  Gain{1..6} (6 alike) : Gain  Gain=RAD2DEG
  log_navigator : ToFile  Filename=./log/SIM/log_navigator.mat  MatrixName=log_navigator  SaveFormat=Timeseries
  quat2eul : MATLAB Function  TreatAsAtomicUnit=on
  wires:
  [log_n_manual_ref] -> Bus Selector/1
  Bus Creator2/1 -> Bus Creator/2  "log_n_offboard_ref"
  Bus Creator/1 -> log_navigator/1  "log_navigator"
  Bus Selector/1 -> Gain3/1  "<euler_ref>"
  Gain3/1 -> Bus Creator1/1  "euler_ref"
  Bus Selector/2 -> Gain1/1  "<rates_ref>"
  Bus Selector/3 -> Bus Creator1/3  "<thrust>"
  Bus Selector/4 -> Bus Creator1/4  "<vel_ref>"
  Bus Creator1/1 -> Bus Creator/1  "log_n_manual_ref"
  Gain1/1 -> Bus Creator1/2  "rates_ref"
  Bus Selector/5 -> Gain2/1  "<delta>"
  Gain2/1 -> Bus Creator1/5  "delta"
  [log_n_offboard_ref] -> Bus Selector1/1  "log_n_offboard_ref"
  Bus Selector1/1 -> Bus Creator2/1  "<pos>"
  Bus Selector1/2 -> Bus Creator2/2  "<vel>"
  Bus Selector1/3 -> Bus Creator2/3  "<acc>"
  Bus Selector1/8 -> Gain4/1  "<rates>"
  Gain4/1 -> Bus Creator2/8  "rates_ref"
  Bus Selector1/9 -> Gain5/1  "<dotrates>"
  Gain5/1 -> Bus Creator2/9  "dotrates"
  quat2eul/1(euler) -> Gain6/1
  Bus Selector1/4 -> Data Type Conversion/1  "<q>"
  Gain6/1 -> Bus Creator2/4  "euler"
  Data Type Conversion/1 -> quat2eul/1(q)
  Bus Selector1/7 -> Bus Creator2/7  "<beta>"
  Bus Selector1/6 -> Bus Creator2/6  "<alpha>"
  Bus Selector1/5 -> Bus Creator2/5  "<f_d>"
  Bus Selector1/10 -> Bus Creator2/10  "<OB_TASK>"

== system LW_ctrl_241029_1/navigator/navigator_offboard/task select ==
  timestamp : Inport
  flight_mode : Inport  Port=2
  pos : Inport  Port=3
  vel : Inport  Port=4
  q : Inport  Port=5
  CH8 : Inport  Port=6
  v_wind : Inport  Port=7
  task select : Subsystem
  offboard_ref : Outport  OutDataTypeStr=Bus: offboard_bus
  wires:
  timestamp/1 -> task select/1(timestamp)
  flight_mode/1 -> task select/2(flight_mode)
  pos/1 -> task select/3(pos)
  vel/1 -> task select/4(vel)
  q/1 -> task select/5(q)
  CH8/1 -> task select/7(CH8)
  task select/1(task1) -> offboard_ref/1
  v_wind/1 -> task select/6(v_wind)

== system LW_ctrl_241029_1/rc_receive/manual_ctrl_in/HIL&FLY V1.13.3 ==
  Bus Creator : BusCreator  Inputs=9
  MATLAB Function : MATLAB Function  TreatAsAtomicUnit=on
  input_rc : pixhawk_slib_sensors_actuators/input_rc  Description=|  sampletime=-1  channel1=on  channel2=on  channel3=on  channel4=on  channel5=on  channel6=on  channel7=on  channel8=on  channel9=off  channel10=off  channel11=off  channel12=off  channel13=off  channel14=off  channel15=off  channel16=off  channel17=off  channel18=off  ch_count=off  rssi=off  rc_failsafe=on  rc_lost=on  rc_inputsource=off
      | RC Input Block
      | 
      | This block provides user input control to the model.
      | It uses the input_rc uORB topic.
      | 
      | The user has the ability to choose which channels are available as outputs from this block and also some optional outputs. These include 
      | Channels 1 through 18
      | double data type indicating the PWM value from the controller 
      | measured pulse widths for each of the supported channels 
      | Channel Count 
      | uint32 data type of the number of channels which are detector by the PX4 
      | RC Failsafe 
      | boolean data types indicating that the RC Tx is sending the FailSafe signal (if equipped and properly setup) 
      | explicit failsafe flag: true on TX failure or TX out of range , false otherwise. 
      | Only the true state is reliable, as there are some (PPM) receivers on the market going into failsafe without telling us explicitly. 
      | RC Input Source 
      | Enumeration data type indicating which source the RC input is from. 
      | Valid values are found in the ENUM file: RC_INPUT_SOURCE_ENUM.m 
      |           Enumeration members for class 'RC_INPUT_SOURCE_ENUM':
      |           RCINPUT_SOURCE_UNKNOWN         (0)
      |           RCINPUT_SOURCE_PX4FMU_PPM      (1)
      |           RCINPUT_SOURCE_PX4IO_PPM       (2)
      |           RCINPUT_SOURCE_PX4IO_SPEKTRUM  (3)
      |           RCINPUT_SOURCE_PX4IO_SBUS      (4)
      |           RCINPUT_SOURCE_PX4IO_ST24      (5)
      |           RCINPUT_SOURCE_MAVLINK         (6)
      |           RCINPUT_SOURCE_QURT            (7)
      |           RCINPUT_SOURCE_PX4FMU_SPEKTRUM (8)
      |           RCINPUT_SOURCE_PX4FMU_SBUS     (9)
      |           RCINPUT_SOURCE_PX4FMU_ST24     (10)
      |           RCINPUT_SOURCE_PX4FMU_SUMD     (11)
      |           RCINPUT_SOURCE_PX4FMU_DSM      (12)
      |           RCINPUT_SOURCE_PX4IO_SUMD      (13)
      | 
      | RSSI - Receive signal strength index 
      | receive signal strength indicator (RSSI): < 0: Undefined, 0: no signal, 255: full reception 
      | RC Lost Connection 
      | boolean data type indicating RC receiver connection status 
      | True, if no frame has arrived in the expected time, false otherwise. 
      | True usally means that the receiver has been disconnected, but can also indicate a radio link loss on "stupid" systems. 
      | Will remain false, if a RX with failsafe option continues to transmit frames after a link loss. 
      |   
      | Sample Model: px4demo_input_rc.slx
      settings: SourceProductName=Sensors and Actuators
  logger : Subsystem  VariantControl=VSS_PROCEDURE_HIL_FLY
  manual_ctrl_in : Outport
  tag scope: log_man=global
  wires:
  input_rc/1 -> MATLAB Function/1(ch1)
  MATLAB Function/2(y) -> Bus Creator/2  "y"
  MATLAB Function/6(AU6) -> Bus Creator/6  "AU6"
  input_rc/7 -> MATLAB Function/7(ch7)
  MATLAB Function/4(r) -> Bus Creator/4  "r"
  input_rc/2 -> MATLAB Function/2(ch2)
  MATLAB Function/1(x) -> Bus Creator/1  "x"
  input_rc/4 -> MATLAB Function/4(ch4)
  MATLAB Function/3(z) -> Bus Creator/3  "z"
  input_rc/8 -> MATLAB Function/8(ch8)
  input_rc/3 -> MATLAB Function/3(ch3)
  MATLAB Function/8(AU8) -> Bus Creator/8  "AU8"
  MATLAB Function/5(AU5) -> Bus Creator/5  "AU5"
  MATLAB Function/7(AU7) -> Bus Creator/7  "AU7"
  input_rc/10 -> MATLAB Function/10(rc_lost)
  MATLAB Function/9(RC_LOST) -> Bus Creator/9  "RC_Lost"
  Bus Creator/1 -> [log_man], manual_ctrl_in/1
  input_rc/9 -> MATLAB Function/9(failsafe)
  input_rc/5 -> MATLAB Function/5(ch5)
  input_rc/6 -> MATLAB Function/6(ch6)

== system LW_ctrl_241029_1/rc_receive/manual_ctrl_in/Sim ==
  Manual Variant Source : simulink/Signal Routing/Manual Variant Source  NumChoices=2  LabelModeActiveChoice=V_1
  Simulate RC : Subsystem  Commented=on
  Simulate ref : Subsystem
  joystick : Subsystem
  logger : Subsystem  VariantControl=VSS_PROCEDURE_SIM
  manual_ctrl_in : Outport  VectorParamsAs1DForOutWhenUnconnected=off
  tag scope: log_man_rc=global
  wires:
  joystick/1(manual_ctrl_in) -> Manual Variant Source/2
  Simulate ref/1(manual_ctrl_in) -> Manual Variant Source/1
  Manual Variant Source/1 -> [log_man_rc], manual_ctrl_in/1

== system LW_ctrl_241029_1/state_machine/logger/HIL&FLY ==
  Bus Selector : BusSelector  OutputSignals=flight_mode,ctrl_mode,arm
  Data Type Conversion : DataTypeConversion  Priority=10  OutDataTypeStr=double  SaturateOnIntegerOverflow=off  RndMeth=Floor
  Data Type Conversion1 : DataTypeConversion  Priority=10  OutDataTypeStr=uint8  SaturateOnIntegerOverflow=off  RndMeth=Floor
  Data Type Conversion2 : DataTypeConversion  Priority=10  OutDataTypeStr=uint8  SaturateOnIntegerOverflow=off  RndMeth=Floor
  Data Type Conversion3 : DataTypeConversion  Priority=10  OutDataTypeStr=uint8  SaturateOnIntegerOverflow=off  RndMeth=Floor
  get_delta_t : Subsystem
  hrt_timestamp : MATLAB Function  TreatAsAtomicUnit=on
  uORB Write Advanced1 : pixhawk_slib_uORB_RW/uORB Write Advanced  Ts=0  uORB_AdvtQueue=on  uORB_FieldEnabledArr="0  0  0  1  0  0  0  0  0  0  0"  uORB_Topic_str=0  uORB_Struct_DT="[1  1  1  1  1]"  BlockInputCount=5  uORB_StructParams="[\"voltage_v\",\"voltage_filtered_v\",\"current_a\",\"current_filtered_a\",\"remaining\"]"  uORB_PortSizes="[1  1  1  1]"  MsgSizeOf=0  MW_update=true
      settings: SourceProductName=uORB Read / Write Blocks
  wires:
  hrt_timestamp/1(ts) -> Data Type Conversion/1
  Data Type Conversion/1 -> uORB Write Advanced1/1, get_delta_t/1(timestamp)
  get_delta_t/1(delta_t) -> uORB Write Advanced1/2
  Bus Selector/2 -> Data Type Conversion2/1  "<ctrl_mode>"
  Data Type Conversion1/1 -> uORB Write Advanced1/3
  Data Type Conversion2/1 -> uORB Write Advanced1/4
  [log_sm_vehicle_mode] -> Bus Selector/1
  Bus Selector/1 -> Data Type Conversion1/1  "<flight_mode>"
  Bus Selector/3 -> Data Type Conversion3/1  "<arm>"
  Data Type Conversion3/1 -> uORB Write Advanced1/5

== system LW_ctrl_241029_1/state_machine/logger/Sim ==
  Bus Creator : BusCreator  Inputs=1
  log_stateMachine : ToFile  Filename=./log/SIM/log_stateMachine.mat  MatrixName=log_stateMachine  SaveFormat=Timeseries
  wires:
  [log_sm_vehicle_mode] -> Bus Creator/1  "log_sm_vehicle_mode"
  Bus Creator/1 -> log_stateMachine/1
